simulink model "poles_step_response"  (R2021a)
settings: Solver=VariableStepAuto  StartTime=0.0  StopTime=10.0  RelTol=1e-3
values from neighbouring files (symbols this model uses):
  B = 20000    [lab2.m]
  J = 600000    [lab2.m]
settings Model: Creator=LEGION  LastModifiedBy=LEGION

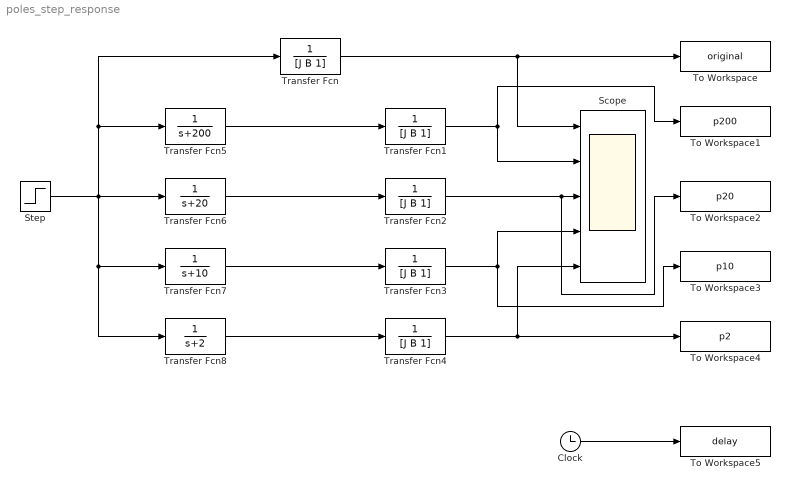
== system poles_step_response ==
  Clock : Clock
  Scope : Scope  NumInputPorts=5
  Step : Step  SampleTime=0
  To Workspace : ToWorkspace  VariableName=original  SaveFormat=Timeseries
  To Workspace1 : ToWorkspace  VariableName=p200  SaveFormat=Timeseries
  To Workspace2 : ToWorkspace  VariableName=p20  SaveFormat=Timeseries
  To Workspace3 : ToWorkspace  VariableName=p10  SaveFormat=Timeseries
  To Workspace4 : ToWorkspace  VariableName=p2  SaveFormat=Timeseries
  To Workspace5 : ToWorkspace  VariableName=delay  SaveFormat=Timeseries
  Transfer Fcn{,1..4} (5 alike) : TransferFcn  Denominator=[J B 1]
  Transfer Fcn5 : TransferFcn  Denominator=[1 200]
  Transfer Fcn6 : TransferFcn  Denominator=[1 20]
  Transfer Fcn7 : TransferFcn  Denominator=[1 10]
  Transfer Fcn8 : TransferFcn  Denominator=[1 2]
  wires:
  Step/1 -> Transfer Fcn8/1, Transfer Fcn7/1, Transfer Fcn/1, Transfer Fcn5/1, Transfer Fcn6/1
  Transfer Fcn5/1 -> Transfer Fcn1/1
  Transfer Fcn6/1 -> Transfer Fcn2/1
  Transfer Fcn7/1 -> Transfer Fcn3/1
  Transfer Fcn8/1 -> Transfer Fcn4/1
  Transfer Fcn/1 -> To Workspace/1, Scope/1
  Transfer Fcn1/1 -> Scope/2, To Workspace1/1
  Transfer Fcn2/1 -> To Workspace2/1, Scope/3
  Transfer Fcn3/1 -> To Workspace3/1, Scope/4
  Transfer Fcn4/1 -> To Workspace4/1, Scope/5
  Clock/1 -> To Workspace5/1
